simulink model "ODE_Hand_Model_v06_gravity_compensation"  (Simulink 7.5)
settings: Solver=ode1  StartTime=0.0  StopTime=inf  FixedStep=0.0315/(3*12)  RelTol=1e-3
settings Model: Creator=nihil  LastModifiedBy=konstantinos

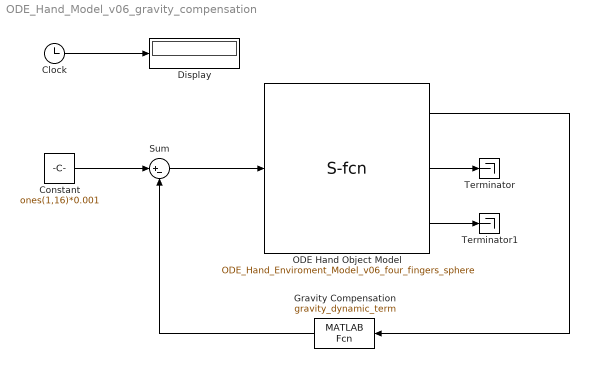
== system ODE_Hand_Model_v06_gravity_compensation ==
  Clock : Clock
      settings: Decimation=10
  Constant : Constant  Value=ones(1,16)*0.001  OutDataType=fixdt(1, 16)  OutScaling=2^0
  Display : Display
  Gravity Compensation : MATLABFcn  MATLABFcn=gravity_dynamic_term
  ODE Hand Object Model : S-Function  FunctionName=ODE_Hand_Enviroment_Model_v06_four_fingers_sphere  EnableBusSupport=off
  Sum : Sum  Inputs=|+-  OutDataType=fixdt(1, 16)  OutScaling=2^0
  Terminator : Terminator
  Terminator1 : Terminator
  wires:
  Clock/1 -> Display/1
  ODE Hand Object Model/2 -> Terminator/1
  ODE Hand Object Model/3 -> Terminator1/1
  ODE Hand Object Model/1 -> Gravity Compensation/1
  Gravity Compensation/1 -> Sum/2
  Constant/1 -> Sum/1
  Sum/1 -> ODE Hand Object Model/1
